simulink model "s1216_91"  (R2019b)
settings: Solver=VariableStepAuto  StartTime=0.0  StopTime=1000  RelTol=1e-3
settings Model: Creator=Administrator  LastModifiedBy=Administrator
settings DebuggingCC: ArithmeticOperatorsInVariantConditions=warning
settings SFSimCC: CustomCodeUndefinedFunction=UseInterfaceOnly

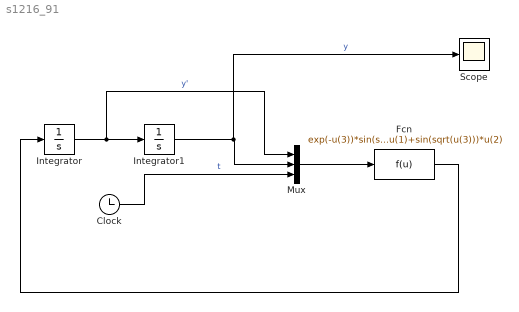
== system s1216_91 ==
  Clock : Clock
  Fcn : Fcn  Expr=exp(-u(3))*sin(sqrt(u(3)))-exp(-(u(3)))*u(1)+sin(sqrt(u(3)))*u(2)
  Integrator : Integrator  InitialCondition=-2
  Integrator1 : Integrator  InitialCondition=1  ZeroCross=off
  Mux : Mux  Inputs=3
  Scope : Scope
  wires:
  Integrator/1 -> Mux/1, Integrator1/1  "y'"
  Integrator1/1 -> Scope/1, Mux/2  "y"
  Clock/1 -> Mux/3  "t"
  Mux/1 -> Fcn/1
  Fcn/1 -> Integrator/1
